simulink model "exp_5"  (R2020a)
settings: Solver=VariableStepAuto  StartTime=0.0  StopTime=10.0  RelTol=1e-3
settings Model: Creator=hp  LastModifiedBy=hp

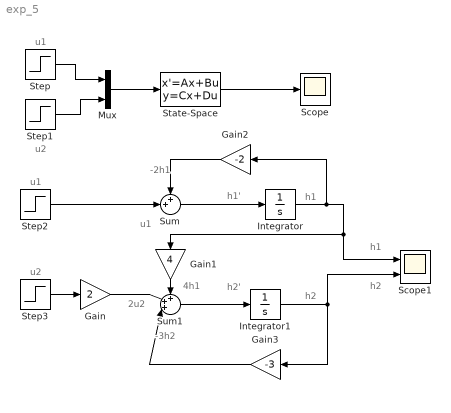
== system exp_5 ==
  note: u1
  note: h1'
  note: h1
  note: h2'
  note: h2
  note: u2
  note: 2u2
  note: 4h1
  note: -3h2
  note: -2h1
  note: u1
  note: h1
  note: h2
  note: u1
  note: u2
  Gain : Gain  Gain=2
  Gain1 : Gain  Gain=4
  Gain2 : Gain  Gain=-2
  Gain3 : Gain  Gain=-3
  Integrator : Integrator
  Integrator1 : Integrator
  Mux : Mux  Inputs=2
  Scope : Scope
  Scope1 : Scope  NumInputPorts=2
  State-Space : StateSpace  A=[-2 0; 4 -3]  B=[1 0; 0 2]  C=[0 1]  D=[0 0]  InitialCondition=0
  Step : Step  SampleTime=0
  Step1 : Step  SampleTime=0
  Step2 : Step  Time=0  SampleTime=0
  Step3 : Step  Time=0  SampleTime=0
  Sum : Sum  Inputs=++|
  Sum1 : Sum  Inputs=+++|
  wires:
  Step/1 -> Mux/1
  Step1/1 -> Mux/2
  Mux/1 -> State-Space/1
  State-Space/1 -> Scope/1
  Step2/1 -> Sum/2
  Integrator/1 -> Scope1/1, Gain1/1, Gain2/1
  Sum/1 -> Integrator/1
  Gain2/1 -> Sum/1
  Gain1/1 -> Sum1/1
  Step3/1 -> Gain/1
  Integrator1/1 -> Scope1/2, Gain3/1
  Gain3/1 -> Sum1/3
  Sum1/1 -> Integrator1/1
  Gain/1 -> Sum1/2
